simulink model "Simple_Model_Packaging_7"  (R2024a)
settings: Solver=VariableStepAuto  StartTime=0.0  StopTime=0.004  RelTol=1e-3
InitFcn:
  | Parameter_Initialize_7
undefined symbols (not defined in the file or in its folder): b, gcbh, ISDFJ_parameter, magnitude, model, n, rcfiltgaincompat, Signal_delay_length, tao, Ts
libraries: simulink x9, commdigbbndfm2 x3, commsink2 x2, commdigbbndam3 x2, commfilt2 x2, commrandsrc3 x2, commchan3 x1, commrfcorlib x1, dspsigops x1, commdigbbndcpm2 x1, commseqgen3 x1, commutil2 x1
(part 1 of 2)
settings Model: Creator=89778  LastModifiedBy=89778
settings OptimizationCC: ReuseModelBlockBuffer=off
settings RTWCC: GPUComputeCapability=3.5

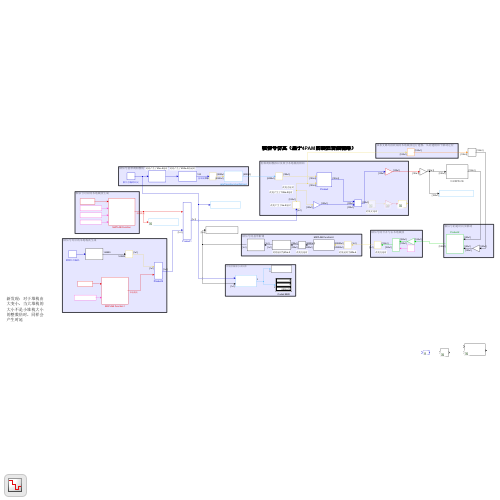
[thumbnail: Simulink's stored preview of the top-level diagram]
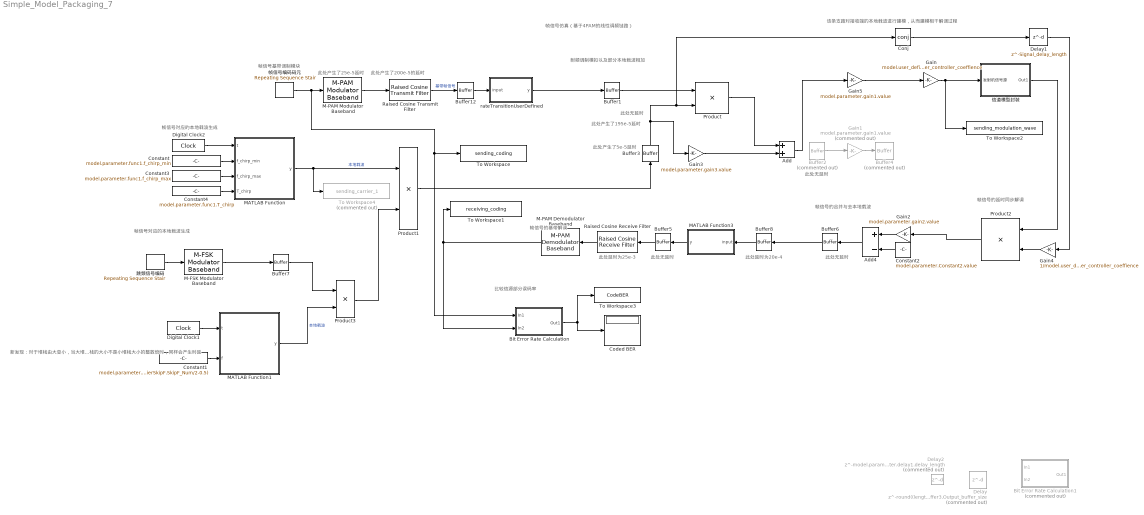
== system Simple_Model_Packaging_7 ==
  note: 帧信号的合并与去本地载波
  note: 帧信号的延时同步解调
  note: 帧信号仿真（基于4PAM的线性调频链路）
  note: 新发现：对于堆栈由大变小，当大堆栈的大小不是小堆栈大小的整数倍时，同样会产生时延
  note: 此处无延时
  note: 此处产生了25e-5延时
  note: 帧信号基带调制模块
  note: 此处产生了200e-5的延时
  note: 帧信号对应的本地载波生成
  note: 此处产生了195e-5延时
  note: 射频调制模拟以及部分本地载波相加
  note: 此处产生了5e-5延时
  note: 此处无延时
  note: 此处无延时
  note: 此处无延时
  note: 此处延时为25e-3
  note: 帧信号的基带解调
  note: 此处延时为20e-4
  note: 该条支路对接收端的本地载波进行建模，从而建模相干解调过程
  note: 比较信源部分误码率
  note: 帧信号对应的本地载波生成
  Add : Sum
  Add4 : Sum  Inputs=+-
  Bit Error Rate Calculation : Subsystem
      mask Display:
      | disp('Bit Error\nRate\nCalculation')
      | port_label('input', 1, 'Tx')
      | port_label('input', 2, 'Rx')
  Bit Error Rate Calculation1 : Subsystem  Commented=on
      mask Display:
      | disp('Bit Error\nRate\nCalculation')
      | port_label('input', 1, 'Tx')
      | port_label('input', 2, 'Rx')
  Buffer1 : Buffer  N=model.parameter.Buffer1.Output_buffer_size  OutputFrames=off
  Buffer12 : Buffer  N=model.parameter.Buffer12.Output_buffer_size  OutputFrames=off
  Buffer2 : Buffer  Commented=on  N=model.parameter.Buffer2.Output_buffer_size  OutputFrames=off
  Buffer3 : Buffer  N=model.parameter.Buffer3.Output_buffer_size  OutputFrames=off
  Buffer4 : Buffer  Commented=on  N=model.parameter.Buffer4.Output_buffer_size  OutputFrames=off
  Buffer5 : Buffer  N=model.parameter.Buffer5.Output_buffer_size  OutputFrames=off
  Buffer6 : Buffer  N=model.parameter.Buffer6.Output_buffer_size  OutputFrames=off
  Buffer7 : Buffer  N=1  OutputFrames=off
  Buffer8 : Buffer  N=model.parameter.Buffer8.Output_buffer_size  OutputFrames=off
  Coded BER : Display
  Conj : Math  Operator=conj
  Constant : Constant  Value=model.parameter.func1.f_chirp_min
  Constant1 : Constant  Value=model.parameter.CarrierSkipF.SkipF_distance*(model.parameter.CarrierSkipF.SkipF_Num/2-0.5)
  Constant2 : Constant  Value=model.parameter.Constant2.value
  Constant3 : Constant  Value=model.parameter.func1.f_chirp_max
  Constant4 : Constant  Value=model.parameter.func1.T_chirp
  Delay : Delay  Commented=on  DelayLength=round((length(model.Parameters.NoiseGen.noise_filter_b)-1)/2)-model.parameter.Buffer3.Output_buffer_size  InitialCondition=0
  Delay1 : Delay  DelayLength=Signal_delay_length  InitialCondition=0
  Delay2 : Delay  Commented=on  DelayLength=model.parameter.delay1.delay_length  InitialCondition=0  InputProcessing=Columns as channels (frame based)
  Digital Clock1 : DigitalClock  SampleTime=model.parameter.Digital_Clock2.CarrierTs
  Digital Clock2 : DigitalClock  SampleTime=model.parameter.Digital_Clock2.CarrierTs
  Gain : Gain  Gain=model.user_defined.TR.Sig_power_controller_coeffience
  Gain1 : Gain  Commented=on  Gain=model.parameter.gain1.value
  Gain2 : Gain  Gain=model.parameter.gain2.value
  Gain3 : Gain  Gain=model.parameter.gain3.value
  Gain4 : Gain  Gain=1/model.user_defined.TR.Sig_power_controller_coeffience
  Gain5 : Gain  Gain=model.parameter.gain1.value
  M-FSK Modulator Baseband : commdigbbndfm2/M-FSK Modulator Baseband  M=model.parameter.CarrierSkipF.SkipF_Num  InType=Integer  Enc=Binary  freqSep=model.parameter.CarrierSkipF.SkipF_distance  phaseType=Continuous  numSamp=ceil(model.parameter.CarrierSkipF.SkipF_time/model.parameter.Repeating_Sequence_Stair.CodeTs)*model.parameter.Raised_Cosine_Transmit_Filter.Output_samples_per_symbol  RateOptions=Enforce single-rate processing  outDataType=double
  M-PAM Demodulator Baseband : commdigbbndam3/M-PAM Demodulator Baseband  M=model.parameter.Rectangular_PAN_Demodulator_Baseband.M_Number  OutType=Integer  Dec=Gray  PowType=Min. distance between symbols  MinDist=model.parameter.Rectangular_PAM_Demodulator_Baseband.Minimum_distance  AvgPow=1  PeakPow=1  outDtype1=Inherit via internal rule  outDtype2=Inherit via internal rule  denormFactorWordLen=16  denormFactorDataTypeStr=Inherit: Same word length as input  denormFactorLastDataTypeStr=Inherit: Same word length as input  prodOutWordLen=16  prodOutRoundingMode=Floor  prodOutOverflowMode=Wrap  prodOutOvFlMode=off  prodOutOvFlModeLastStrValue=off  sumWordLen=16
  M-PAM Modulator Baseband : commdigbbndam3/M-PAM Modulator Baseband  M=model.parameter.M_PAM_Modulator_Baseband.M_ary_number  InType=Integer  Enc=Gray  PowType=Min. distance between symbols  MinDist=model.parameter.M_PAM_Modulator_Baseband.Minimum_distance  AvgPow=1  PeakPow=1  outDtype=double  outWordLen=16  outUDDataType=sfix(16)  outFracLenMode=Best precision  outFracLen=15  outDataTypeStr=double  outLastDataTypeStr=double
  MATLAB Function : MATLAB Function  InitFcn=|  TreatAsAtomicUnit=on
      | f_chirp_min=4.8e6;
      | f_chirp_max=5.2e6;
      | T_chirp=4e-4;
  MATLAB Function1 : MATLAB Function  InitFcn=|  TreatAsAtomicUnit=on
      | f_chirp_min=4.8e6;
      | f_chirp_max=5.2e6;
      | T_chirp=4e-4;
  MATLAB Function3 : MATLAB Function  TreatAsAtomicUnit=on
  Product{,1..3} (4 alike) : Product
  Raised Cosine Receive Filter : commfilt2/Raised Cosine Receive Filter  filtType=Square root  R=model.parameter.Raised_Cosine_Receive_Filter.Rolloff_factor  filtSpan=model.parameter.Raised_Cosine_Receive_Filter.Filter_span_in_symbols  N=model.parameter.Raised_Cosine_Receive_Filter.Input_samples_per_symbol  downFactor=model.parameter.Raised_Cosine_Receive_Filter.Decimation_factor  downOffset=0  filterGain=rcfiltgaincompat(gcbh)  InputProcessing=Columns as channels (frame based)  RateOptions=Enforce single-rate processing  framing=Mute  checkCoeff=off  variableName=rcRxFilt  currentFiltSpan=10  D=5  inputOffset=0  sampMode=Mute  saveAsFlag=0  rateMode=Downsampling  checkGain=Normalized  launchFVT=on  roundingMode=Floor  overflowMode=off  coeffDataTypeStr=Inherit: Same word length as input  coeffMin=[]  coeffMax=[]  coeffLastDataTypeStr=Inherit: Same word length as input  accumDataTypeStr=Inherit: Same as product output  accumLastDataTypeStr=Inherit: Same as product output  outputDataTypeStr=Inherit: Same as accumulator  outputMin=[]  outputMax=[]  outputLastDataTypeStr=Inherit: Same as accumulator
  Raised Cosine Transmit Filter : commfilt2/Raised Cosine Transmit Filter  filtType=Square root  R=model.parameter.Raised_Cosine_Transmit_Filter.Rolloff_factor  filtSpan=model.parameter.Raised_Cosine_Transmit_Filter.Filter_span_in_symbols  N=model.parameter.Raised_Cosine_Transmit_Filter.Output_samples_per_symbol  filterGain=rcfiltgaincompat(gcbh)  InputProcessing=Columns as channels (frame based)  RateOptions=Enforce single-rate processing  framing=Mute  checkCoeff=off  variableName=rcTxFilt  checkGain=Normalized  sampMode=Mute  saveAsFlag=0  currentFiltSpan=10  D=(10)/2  launchFVT=on  roundingMode=Floor  overflowMode=off  coeffDataTypeStr=Inherit: Same word length as input  coeffMin=[]  coeffMax=[]  coeffLastDataTypeStr=Inherit: Same word length as input  outputDataTypeStr=Inherit: Same as accumulator  outputMin=[]  outputMax=[]  outputLastDataTypeStr=Inherit: Same as accumulator
  To Workspace : ToWorkspace  VariableName=sending_coding  SaveFormat=Timeseries  SampleTime=-1
  To Workspace1 : ToWorkspace  VariableName=receiving_coding  SaveFormat=Timeseries  SampleTime=-1
  To Workspace2 : ToWorkspace  VariableName=sending_modulation_wave  SaveFormat=Timeseries  SampleTime=-1
  To Workspace3 : ToWorkspace  VariableName=CodeBER  SaveFormat=Timeseries  SampleTime=-1
  To Workspace4 : ToWorkspace  Commented=on  VariableName=sending_carrier_1  SaveFormat=Timeseries  SampleTime=-1
  rateTransitionUserDefined : MATLAB Function  TreatAsAtomicUnit=on
  信道模型封装 : Subsystem
  帧信号编码码元 : simulink/Sources/Repeating Sequence Stair  OutValues=model.parameter.Repeating_Sequence_Stair.output_vector  tsamp=model.parameter.Repeating_Sequence_Stair.CodeTs  OutMin=[]  OutMax=[]  OutDataTypeStr=double  OutputDataTypeScalingMode=double  OutDataType=fixdt(0,8)  ConRadixGroup=Best Precision: Vector-wise  OutScaling=2^-12
  跳频信号编码 : simulink/Sources/Repeating Sequence Stair  OutValues=model.parameter.CarrierSkipF.SkipF_vector  tsamp=model.parameter.Digital_Clock2.CarrierTs*ceil(model.parameter.CarrierSkipF.SkipF_time/model.parameter.Repeating_Sequence_Stair.CodeTs)*model.parameter.Raised_Cosine_Transmit_Filter.Output_samples_per_symbol  OutMin=[]  OutMax=[]  OutDataTypeStr=double  OutputDataTypeScalingMode=double  OutDataType=fixdt(0,8)  ConRadixGroup=Best Precision: Vector-wise  OutScaling=2^-12
  wires:
  Buffer2/1 -> Gain1/1
  Buffer12/1 -> rateTransitionUserDefined/1(input)
  rateTransitionUserDefined/1(y) -> Buffer1/1
  Raised Cosine Transmit Filter/1 -> Buffer12/1  "基带帧信号"
  M-PAM Modulator Baseband/1 -> Raised Cosine Transmit Filter/1
  Digital Clock2/1 -> MATLAB Function/1(t)
  Buffer1/1 -> Product/1
  Gain1/1 -> Buffer4/1
  Buffer5/1 -> Raised Cosine Receive Filter/1
  MATLAB Function3/1(y) -> Buffer5/1
  Buffer8/1 -> MATLAB Function3/1(input)
  Buffer6/1 -> Buffer8/1
  Raised Cosine Receive Filter/1 -> M-PAM Demodulator Baseband/1
  Constant/1 -> MATLAB Function/2(f_chirp_min)
  Constant3/1 -> MATLAB Function/3(f_chirp_max)
  Constant4/1 -> MATLAB Function/4(T_chirp)
  Gain/1 -> To Workspace2/1, 信道模型封装/1(发射机信号源)
  Gain4/1 -> Product2/2
  信道模型封装/1(Out1) -> Product2/1
  Gain3/1 -> Add/2
  Product/1 -> Add/1
  Buffer3/1 -> Gain3/1, Conj/1, Product/2
  Gain2/1 -> Add4/1
  Constant2/1 -> Add4/2
  Product2/1 -> Gain2/1
  Add4/1 -> Buffer6/1
  Add/1 -> Gain5/1
  Gain5/1 -> Gain/1
  跳频信号编码/1 -> M-FSK Modulator Baseband/1
  MATLAB Function/1(y) -> Product1/1, To Workspace4/1  "本地载波"
  Product1/1 -> Buffer3/1
  M-FSK Modulator Baseband/1 -> Buffer7/1
  Constant1/1 -> MATLAB Function1/2(f)
  Digital Clock1/1 -> MATLAB Function1/1(t)
  Buffer7/1 -> Product3/1
  MATLAB Function1/1(y) -> Product3/2  "本地载波"
  Product3/1 -> Product1/2
  M-PAM Demodulator Baseband/1 -> Bit Error Rate Calculation/2(In2), To Workspace1/1
  Bit Error Rate Calculation/1(Out1) -> Coded BER/1, To Workspace3/1
  Conj/1 -> Delay1/1
  Delay1/1 -> Gain4/1
  帧信号编码码元/1 -> Bit Error Rate Calculation/1(In1), To Workspace/1, M-PAM Modulator Baseband/1

== system Simple_Model_Packaging_7/Bit Error Rate Calculation ==
  In1 : Inport
  In2 : Inport  Port=2
  Error Rate Calculation : commsink2/Error Rate Calculation  N=920 + Signal_delay_length*4  st_delay=0  cp_mode=Entire frame  subframe=[]  PMode=Port  WsName=ErrorVec  RsMode2=off  stop=on  numErr=1e8  maxBits=1e10
  Integer to Bit Converter : simulink/Logic and Bit Operations/Integer to Bit Converter  nbits=4  signedInputValues=Unsigned  bitOrder=MSB first  outDtype=Inherit via internal rule
      settings: LibrarySourceBlock=|
      | commutil2/Integer to Bit
      | Converter
  Integer to Bit Converter1 : simulink/Logic and Bit Operations/Integer to Bit Converter  nbits=4  signedInputValues=Unsigned  bitOrder=MSB first  outDtype=Inherit via internal rule
      settings: LibrarySourceBlock=|
      | commutil2/Integer to Bit
      | Converter
  Out1 : Outport  VectorParamsAs1DForOutWhenUnconnected=off
  wires:
  Integer to Bit Converter/1 -> Error Rate Calculation/1
  Integer to Bit Converter1/1 -> Error Rate Calculation/2
  In1/1 -> Integer to Bit Converter/1
  Error Rate Calculation/1 -> Out1/1
  In2/1 -> Integer to Bit Converter1/1

== system Simple_Model_Packaging_7/Bit Error Rate Calculation1 ==
  In1 : Inport
  In2 : Inport  Port=2
  Error Rate Calculation : commsink2/Error Rate Calculation  N=920 + 4*round((length(model.Parameters.NoiseGen.noise_filter_b)-1)/2)  st_delay=0  cp_mode=Entire frame  subframe=[]  PMode=Port  WsName=ErrorVec  RsMode2=off  stop=on  numErr=1e8  maxBits=1e10
  Integer to Bit Converter : simulink/Logic and Bit Operations/Integer to Bit Converter  nbits=4  signedInputValues=Unsigned  bitOrder=MSB first  outDtype=Inherit via internal rule
      settings: LibrarySourceBlock=|
      | commutil2/Integer to Bit
      | Converter
  Integer to Bit Converter1 : simulink/Logic and Bit Operations/Integer to Bit Converter  nbits=4  signedInputValues=Unsigned  bitOrder=MSB first  outDtype=Inherit via internal rule
      settings: LibrarySourceBlock=|
      | commutil2/Integer to Bit
      | Converter
  Out1 : Outport  VectorParamsAs1DForOutWhenUnconnected=off
  wires:
  Integer to Bit Converter/1 -> Error Rate Calculation/1
  Integer to Bit Converter1/1 -> Error Rate Calculation/2
  In1/1 -> Integer to Bit Converter/1
  Error Rate Calculation/1 -> Out1/1
  In2/1 -> Integer to Bit Converter1/1

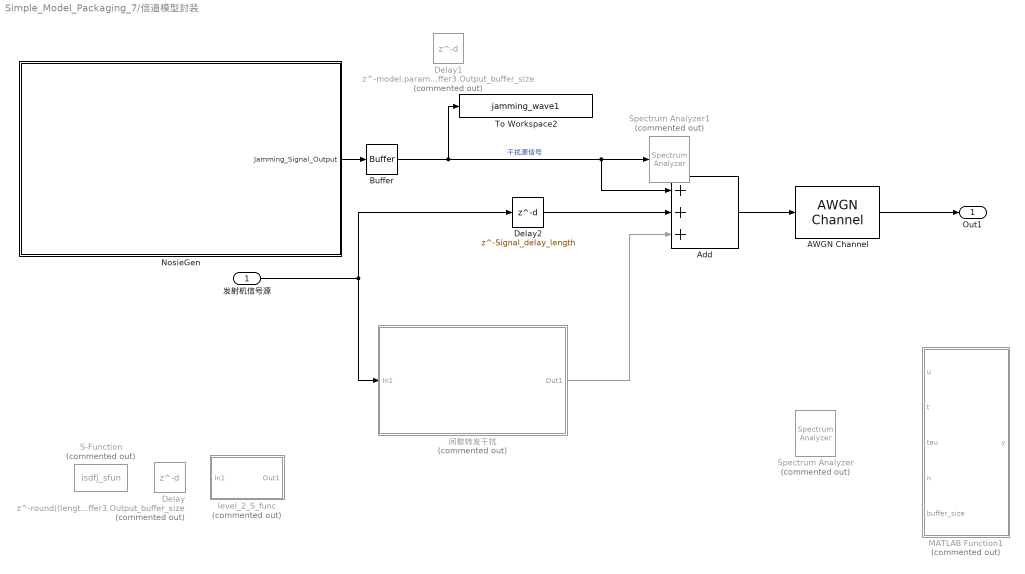
== system Simple_Model_Packaging_7/信道模型封装 ==
  发射机信号源 : Inport
  AWGN Channel : commchan3/AWGN Channel  LegacyMode=on  NoiseMethod="Signal to noise ratio  (SNR)"  noiseMode="Signal to noise ratio  (SNR)"  EbNo=10  EsNo=10  SNR=model.parameter.Awgn.SNR  BitsPerSymbol=1  SignalPower=model.parameter.Awgn.input_power  SamplesPerSymbol=1  SymbolPeriod=1  VarianceSource=Parameter  Variance=1  RandomStream=Global stream  Seed=67  SimulateUsing=Code generation
  Add : Sum  Inputs=+++
  Buffer : Buffer  N=model.parameter.Buffer1.Output_buffer_size  OutputFrames=off
  Delay : Delay  Commented=on  DelayLength=round((length(model.Parameters.NoiseGen.noise_filter_b)-1)/2)-model.parameter.Buffer3.Output_buffer_size  InitialCondition=0
  Delay1 : Delay  Commented=on  DelayLength=model.parameter.Buffer3.Output_buffer_size  InitialCondition=0
  Delay2 : Delay  DelayLength=Signal_delay_length  InitialCondition=0
  MATLAB Function1 : MATLAB Function  Commented=on  TreatAsAtomicUnit=on
  NosieGen : Subsystem
  S-Function : S-Function  Commented=on  FunctionName=isdfj_sfun  Parameters=tao,Ts,n  SFunctionDeploymentMode=off  EnableBusSupport=off
  Spectrum Analyzer : SpectrumAnalyzer  Commented=on  WindowPosition=[81 208 916 450]  SampleRate=285714285.714286  AxesScaling=Manual  Span=285714285.714286  StartFrequency=-142857142.857143  StopFrequency=142857142.857143  AveragingMethod=Exponential  YLimits=[-69.74794186129295781,48.725459434063161268]  AllowFFTLengthLessThanSamplesPerUpdate=on
  Spectrum Analyzer1 : SpectrumAnalyzer  Commented=on  WindowPosition=[746 192 916 450]  SampleRate=285714285.714286  AxesScaling=Manual  Span=285714285.714286  StartFrequency=-142857142.857143  StopFrequency=142857142.857143  AveragingMethod=Exponential  YLimits=[16.792703666476541002,24.095744456486141161]  AllowFFTLengthLessThanSamplesPerUpdate=on
  To Workspace2 : ToWorkspace  VariableName=jamming_wave1  SaveFormat=Timeseries  SampleTime=-1
  level_2_S_func : Subsystem  Commented=on
  间歇转发干扰 : Subsystem  Commented=on
  Out1 : Outport
  wires:
  AWGN Channel/1 -> Out1/1
  Add/1 -> AWGN Channel/1
  发射机信号源/1 -> Delay2/1, 间歇转发干扰/1(In1)
  Buffer/1 -> To Workspace2/1, Spectrum Analyzer1/1, Add/1  "干扰源信号"
  NosieGen/1(Jamming_Signal_Output) -> Buffer/1
  Delay2/1 -> Add/2
  间歇转发干扰/1(Out1) -> Add/3

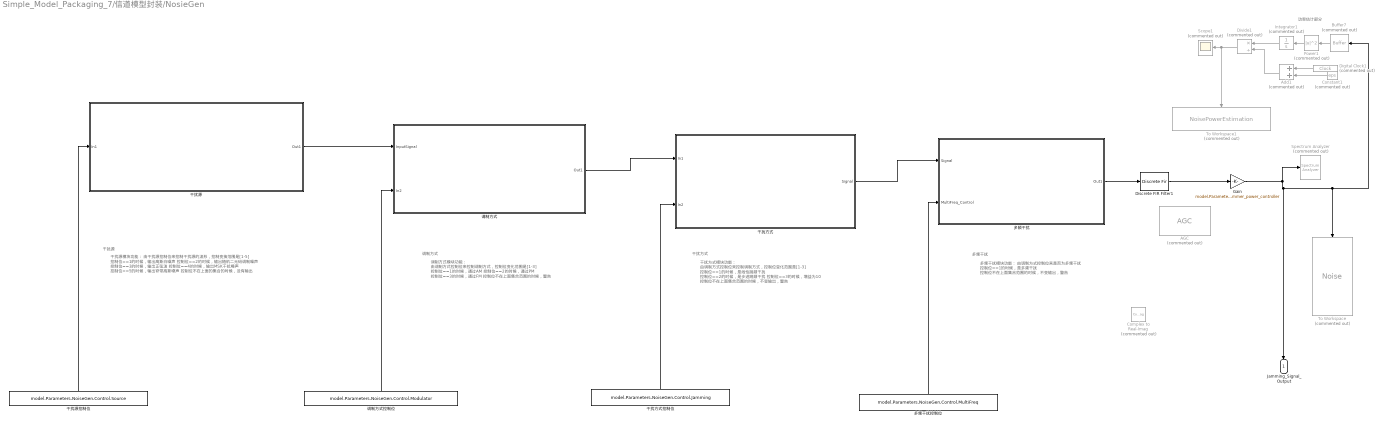
== system Simple_Model_Packaging_7/信道模型封装/NosieGen ==
  note: 调制方式
  note: 调制方式模块功能：
      | 由调制方式控制位来控制调制方式，控制位变化范围是[1-3]
      | 控制位==1的时候，通过AM
      | 控制位==2的时候，通过PM
      | 控制位==3的时候，通过FM
      |
      | 控制位不在上面集合范围的时候，警告
  note: 干扰方式模块功能：
      | 由调制方式控制位来控制调制方式，控制位变化范围是[1-3]
      | 控制位==1的时候，是线性跳频干扰
      | 控制位==2的时候，是步进跳频干扰
      | 控制位==3的时候，增益为10
      |
      | 控制位不在上面集合范围的时候，不变输出，警告
  note: 干扰源
  note: 功率估计部分
  note: 干扰方式
  note: 干扰源模块功能：
      | 由干扰源控制位来控制干扰源的波形，控制变换范围是[1-5]
      | 控制位==1的时候，输出高斯白噪声
      | 控制位==2的时候，输出随机二元码调制噪声
      | 控制位==3的时候，输出正弦波
      | 控制位==4的时候，输出MSK干扰噪声
      | 控制位==5的时候，输出窄带高斯噪声
      | 控制位不在上面的集合的时候，没有输出
  note: 多频干扰模块功能：
      | 由调制方式控制位来是否为多频干扰
      | 控制位==1的时候，是多频干扰
      |
      | 控制位不在上面集合范围的时候，不变输出，警告
  note: 多频干扰
  AGC : commrfcorlib/AGC  Commented=on  LegacyMode=off  DetectorMethod=Rectifier  LoopMethod=Linear  UpdatePeriod=100  StepSize=0.1  AdaptationStepSize=0.01  DesiredOutputPower=1  AveragingLength=100  MaximumGain=30  MaxPowerGain=60  GainOutputPort=off  InputPowerOutputPort=off  SimulateUsing=Interpreted execution
  Add1 : Sum  Commented=on
  Buffer7 : Buffer  Commented=on  N=1  OutputFrames=off
  Complex to Real-Imag : ComplexToRealImag  Commented=on
  Constant1 : Constant  Commented=on  Value=eps  SampleTime=model.Parameters.NoiseGen.NoiseTs
  Digital Clock1 : DigitalClock  Commented=on  SampleTime=model.Parameters.NoiseGen.NoiseTs
  Discrete FIR Filter1 : DiscreteFir  Coefficients=model.Parameters.NoiseGen.noise_filter_b
  Divide1 : Product  Commented=on  Inputs=*/
  Gain : Gain  Gain=model.Parameters.jammer_power_controller
  Integrator1 : Integrator  Commented=on
  Power1 : Math  Commented=on  Operator=magnitude^2
  Scope1 : Scope  Commented=on
  Spectrum Analyzer : SpectrumAnalyzer  Commented=on  WindowPosition=[162 288 916 450]  SampleRate=340000000  AxesScaling=Manual  Span=340000000  StartFrequency=-170000000  StopFrequency=170000000  AveragingMethod=Exponential  YLimits=[16.792703666476541002,24.095744456486141161]  AllowFFTLengthLessThanSamplesPerUpdate=on
  To Workspace : ToWorkspace  Commented=on  VariableName=Noise  SaveFormat=Timeseries  SampleTime=-1
  To Workspace1 : ToWorkspace  Commented=on  VariableName=NoisePowerEstimation  SaveFormat=Timeseries  SampleTime=-1
  多频干扰 : Subsystem
  多频干扰控制位 : Constant  Value=model.Parameters.NoiseGen.Control.MultiFreq  SampleTime=Inf
  干扰方式 : Subsystem
  干扰方式控制位 : Constant  Value=model.Parameters.NoiseGen.Control.Jamming  SampleTime=Inf
  干扰源 : Subsystem
  干扰源控制位 : Constant  Value=model.Parameters.NoiseGen.Control.Source  SampleTime=Inf
  调制方式 : Subsystem
  调制方式控制位 : Constant  Value=model.Parameters.NoiseGen.Control.Modulator  SampleTime=Inf
  Jamming_Signal_Output : Outport
  wires:
  Integrator1/1 -> Divide1/1
  Power1/1 -> Integrator1/1
  干扰方式控制位/1 -> 干扰方式/2(In2)
  调制方式控制位/1 -> 调制方式/2(In2)
  Digital Clock1/1 -> Add1/1
  Divide1/1 -> Scope1/1, To Workspace1/1
  干扰源控制位/1 -> 干扰源/1(In1)
  Constant1/1 -> Add1/2
  Add1/1 -> Divide1/2
  Buffer7/1 -> Power1/1
  Gain/1 -> Jamming_Signal_Output/1, Buffer7/1, To Workspace/1, Spectrum Analyzer/1
  调制方式/1(Out1) -> 干扰方式/1(In1)
  干扰源/1(Out1) -> 调制方式/1(InputSignal)
  多频干扰控制位/1 -> 多频干扰/2(MultiFreq_Control)
  干扰方式/1(Signal) -> 多频干扰/1(Signal)
  多频干扰/1(Out1) -> Discrete FIR Filter1/1
  Discrete FIR Filter1/1 -> Gain/1

== system Simple_Model_Packaging_7/信道模型封装/level_2_S_func ==
  In1 : Inport
  Buffer1 : Buffer  N=1  OutputFrames=off
  Buffer2 : Buffer  N=100  OutputFrames=off
  Level-2 MATLAB S-Function : M-S-Function  FunctionName=isdfj_sfun  Parameters=2e-6, 10e-6, 1
  Out1 : Outport
  wires:
  Level-2 MATLAB S-Function/1 -> Buffer2/1
  Buffer2/1 -> Out1/1
  Buffer1/1 -> Level-2 MATLAB S-Function/1
  In1/1 -> Buffer1/1

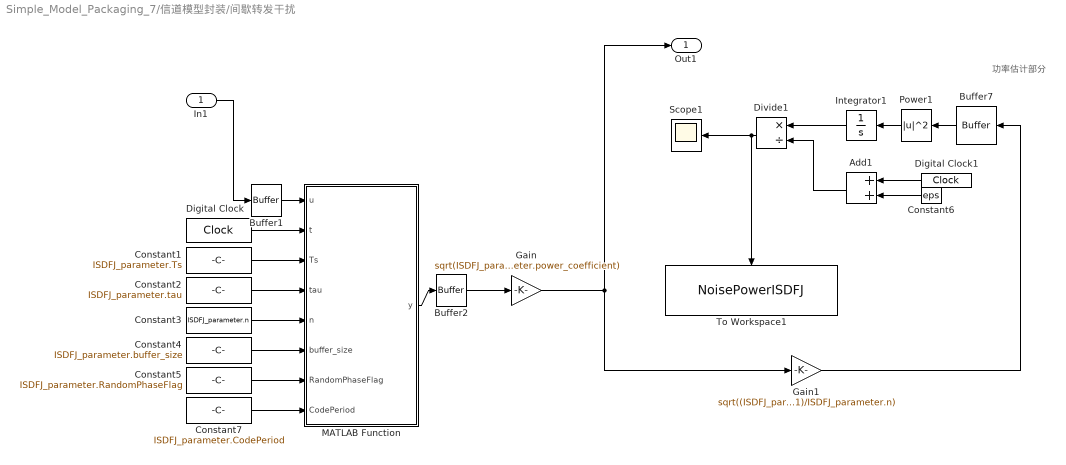
== system Simple_Model_Packaging_7/信道模型封装/间歇转发干扰 ==
  note: 功率估计部分
  In1 : Inport
  Add1 : Sum
  Buffer1 : Buffer  N=1  OutputFrames=off
  Buffer2 : Buffer  N=100  OutputFrames=off
  Buffer7 : Buffer  N=1  OutputFrames=off
  Constant1 : Constant  Value=ISDFJ_parameter.Ts
  Constant2 : Constant  Value=ISDFJ_parameter.tau
  Constant3 : Constant  Value=ISDFJ_parameter.n
  Constant4 : Constant  Value=ISDFJ_parameter.buffer_size
  Constant5 : Constant  Value=ISDFJ_parameter.RandomPhaseFlag
  Constant6 : Constant  Value=eps  SampleTime=model.Parameters.NoiseGen.NoiseTs
  Constant7 : Constant  Value=ISDFJ_parameter.CodePeriod
  Digital Clock : DigitalClock  SampleTime=model.Parameters.NoiseGen.NoiseTs
  Digital Clock1 : DigitalClock  SampleTime=model.Parameters.NoiseGen.NoiseTs
  Divide1 : Product  Inputs=*/
  Gain : Gain  Gain=sqrt(ISDFJ_parameter.power_coefficient)
  Gain1 : Gain  Gain=sqrt((ISDFJ_parameter.n+1)/ISDFJ_parameter.n)
  Integrator1 : Integrator
  MATLAB Function : MATLAB Function  TreatAsAtomicUnit=on
  Power1 : Math  Operator=magnitude^2
  Scope1 : Scope
  To Workspace1 : ToWorkspace  VariableName=NoisePowerISDFJ  SaveFormat=Timeseries  SampleTime=-1
  Out1 : Outport
  wires:
  Constant2/1 -> MATLAB Function/4(tau)
  In1/1 -> Buffer1/1
  Constant1/1 -> MATLAB Function/3(Ts)
  Constant3/1 -> MATLAB Function/5(n)
  Digital Clock/1 -> MATLAB Function/2(t)
  MATLAB Function/1(y) -> Buffer2/1
  Constant4/1 -> MATLAB Function/6(buffer_size)
  Buffer1/1 -> MATLAB Function/1(u)
  Constant5/1 -> MATLAB Function/7(RandomPhaseFlag)
  Power1/1 -> Integrator1/1
  Add1/1 -> Divide1/2
  Buffer7/1 -> Power1/1
  Constant6/1 -> Add1/2
  Integrator1/1 -> Divide1/1
  Digital Clock1/1 -> Add1/1
  Divide1/1 -> Scope1/1, To Workspace1/1
  Constant7/1 -> MATLAB Function/8(CodePeriod)
  Gain/1 -> Out1/1, Gain1/1
  Gain1/1 -> Buffer7/1
  Buffer2/1 -> Gain/1

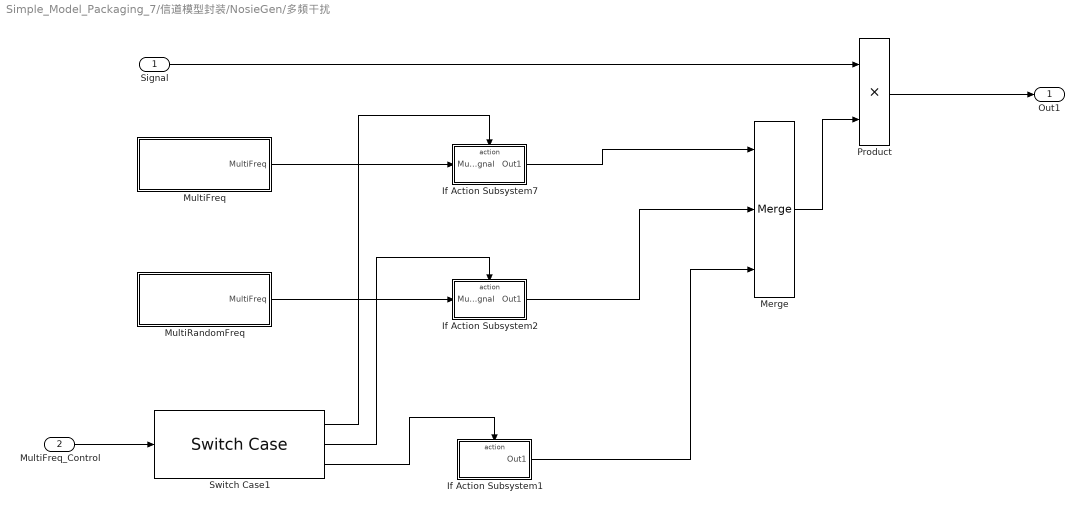
== system Simple_Model_Packaging_7/信道模型封装/NosieGen/多频干扰 ==
  Signal : Inport
  MultiFreq_Control : Inport  Port=2
  If Action Subsystem1 : Subsystem  TreatAsAtomicUnit=on
  If Action Subsystem2 : Subsystem  TreatAsAtomicUnit=on
  If Action Subsystem7 : Subsystem  TreatAsAtomicUnit=on
  Merge : Merge  Inputs=3
  MultiFreq : Subsystem
  MultiRandomFreq : Subsystem
  Product : Product
  Switch Case1 : SwitchCase  CaseConditions={1,2}
  Out1 : Outport
  wires:
  Switch Case1/3 -> If Action Subsystem1/Action
  Signal/1 -> Product/1
  MultiFreq_Control/1 -> Switch Case1/1
  Merge/1 -> Product/2
  Product/1 -> Out1/1
  Switch Case1/1 -> If Action Subsystem7/Action
  MultiFreq/1(MultiFreq) -> If Action Subsystem7/1(MultiFreqSignal)
  If Action Subsystem7/1(Out1) -> Merge/1
  If Action Subsystem1/1(Out1) -> Merge/3
  MultiRandomFreq/1(MultiFreq) -> If Action Subsystem2/1(MultiRandomFreqSignal)
  Switch Case1/2 -> If Action Subsystem2/Action
  If Action Subsystem2/1(Out1) -> Merge/2

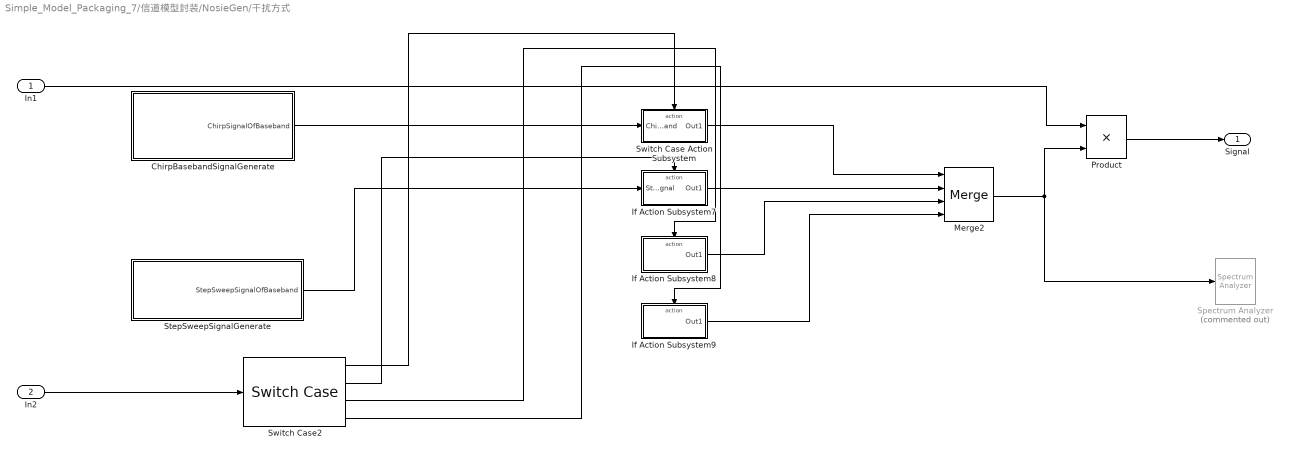
== system Simple_Model_Packaging_7/信道模型封装/NosieGen/干扰方式 ==
  In1 : Inport
  In2 : Inport  Port=2
  ChirpBasebandSignalGenerate : Subsystem
      settings: AttributesFormatString=|
      | 线性调频模块：线性调频公式(y=exp(2*pi*(f_min*t+0.5*k_chirp*t^2)))
      | 输入参数：
      | 1. f_min,为线性调频信号的起始频率
      | 2.f_max为线性调频信号的终止频率
      | 3.T_chirp为线性调频信号的调频时间
      | 斜率k_sweep = (f_min-f_max)/T_chirp
  If Action Subsystem7 : Subsystem  TreatAsAtomicUnit=on
  If Action Subsystem8 : Subsystem  TreatAsAtomicUnit=on
  If Action Subsystem9 : Subsystem  TreatAsAtomicUnit=on
  Merge2 : Merge  Inputs=4
  Product : Product
  Spectrum Analyzer : SpectrumAnalyzer  Commented=on  WindowPosition=[-1041 199 916 450]  SampleRate=340000000  AxesScaling=Manual  Span=340000000  StartFrequency=-170000000  StopFrequency=170000000  AveragingMethod=Exponential  YLimits=[-55.253534235882824532,34.529267970454846193]  AllowFFTLengthLessThanSamplesPerUpdate=on
  StepSweepSignalGenerate : Subsystem
  Switch Case Action Subsystem : Subsystem  TreatAsAtomicUnit=on
  Switch Case2 : SwitchCase  CaseConditions={1,2,3}
  Signal : Outport
  wires:
  If Action Subsystem9/1(Out1) -> Merge2/4
  Switch Case Action Subsystem/1(Out1) -> Merge2/1
  If Action Subsystem8/1(Out1) -> Merge2/3
  Switch Case2/3 -> If Action Subsystem8/Action
  Switch Case2/1 -> Switch Case Action Subsystem/Action
  Switch Case2/2 -> If Action Subsystem7/Action
  Switch Case2/4 -> If Action Subsystem9/Action
  ChirpBasebandSignalGenerate/1(ChirpSignalOfBaseband) -> Switch Case Action Subsystem/1(ChirpSignalOfBaseband)
  If Action Subsystem7/1(Out1) -> Merge2/2
  Merge2/1 -> Spectrum Analyzer/1, Product/2
  Product/1 -> Signal/1
  In1/1 -> Product/1
  In2/1 -> Switch Case2/1
  StepSweepSignalGenerate/1(StepSweepSignalOfBaseband) -> If Action Subsystem7/1(StepSweepSignal)

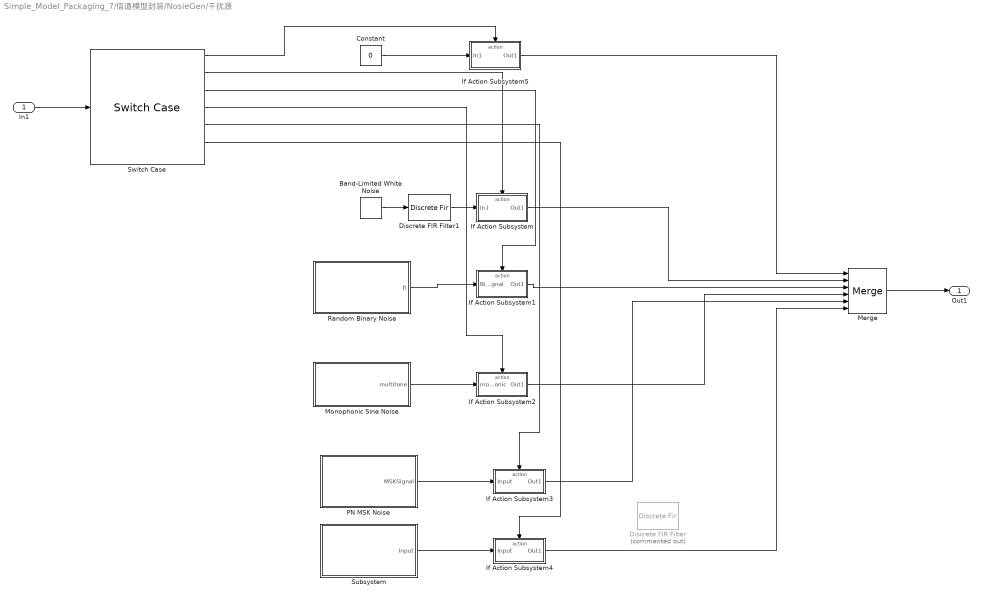
== system Simple_Model_Packaging_7/信道模型封装/NosieGen/干扰源 ==
  In1 : Inport
  Band-Limited White Noise : simulink/Sources/Band-Limited White Noise  Cov=model.Parameters.NoiseGen.GaussPower  Ts=model.Parameters.NoiseGen.NoiseTs  seed=model.Parameters.NoiseGen.GaussSeed
  Constant : Constant  Value=0  SampleTime=model.Parameters.NoiseGen.NoiseTs
  Discrete FIR Filter : DiscreteFir  Commented=on  Coefficients=b
  Discrete FIR Filter1 : DiscreteFir  Coefficients=model.Parameters.NoiseGen.pulse_noise_filter_b
  If Action Subsystem : Subsystem  TreatAsAtomicUnit=on
  If Action Subsystem1 : Subsystem  TreatAsAtomicUnit=on
  If Action Subsystem2 : Subsystem  TreatAsAtomicUnit=on
  If Action Subsystem3 : Subsystem  TreatAsAtomicUnit=on
  If Action Subsystem4 : Subsystem  TreatAsAtomicUnit=on
  If Action Subsystem5 : Subsystem  TreatAsAtomicUnit=on
  Merge : Merge  Inputs=6
  Monophonic Sine Noise : Subsystem
  PN MSK Noise : Subsystem
  Random Binary Noise : Subsystem
  Subsystem : Subsystem
  Switch Case : SwitchCase  CaseConditions={0,1,2,3,4,5}
  Out1 : Outport
  wires:
  Switch Case/3 -> If Action Subsystem1/Action
  If Action Subsystem2/1(Out1) -> Merge/4
  Band-Limited White Noise/1 -> Discrete FIR Filter1/1
  If Action Subsystem1/1(Out1) -> Merge/3
  Random Binary Noise/1(Jt) -> If Action Subsystem1/1(Binary_Random_Signal)
  Switch Case/4 -> If Action Subsystem2/Action
  Switch Case/2 -> If Action Subsystem/Action
  Merge/1 -> Out1/1
  In1/1 -> Switch Case/1
  Monophonic Sine Noise/1(multitone) -> If Action Subsystem2/1(monophonic)
  Switch Case/5 -> If Action Subsystem3/Action
  If Action Subsystem3/1(Out1) -> Merge/5
  If Action Subsystem/1(Out1) -> Merge/2
  PN MSK Noise/1(MSKSignal) -> If Action Subsystem3/1(Input)
  Switch Case/6 -> If Action Subsystem4/Action
  Subsystem/1(Input) -> If Action Subsystem4/1(Input)
  If Action Subsystem4/1(Out1) -> Merge/6
  Switch Case/1 -> If Action Subsystem5/Action
  Constant/1 -> If Action Subsystem5/1(In1)
  If Action Subsystem5/1(Out1) -> Merge/1
  Discrete FIR Filter1/1 -> If Action Subsystem/1(In1)

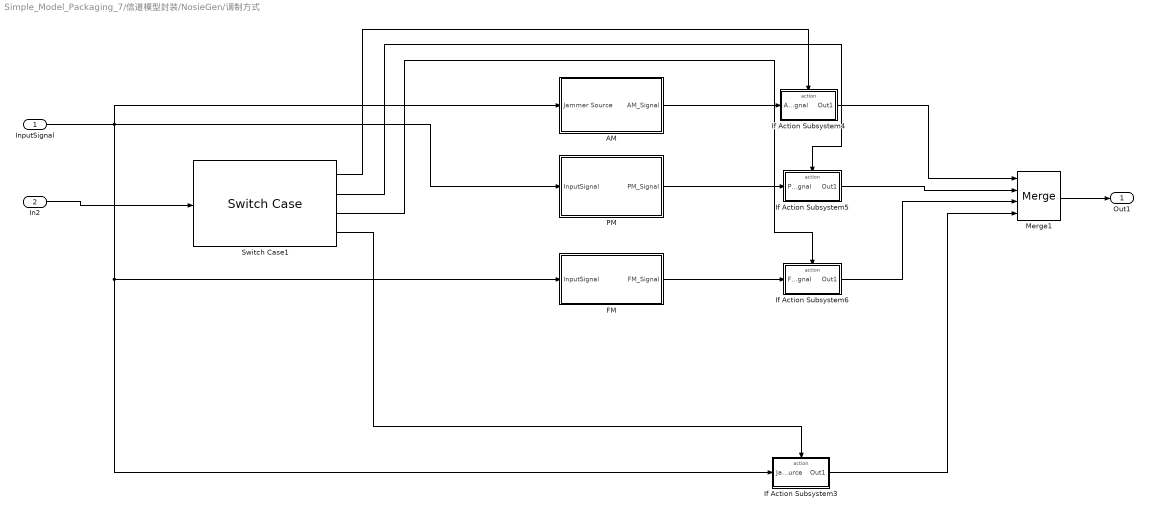
== system Simple_Model_Packaging_7/信道模型封装/NosieGen/调制方式 ==
  InputSignal : Inport
  In2 : Inport  Port=2
  AM : Subsystem
  FM : Subsystem
  If Action Subsystem3 : Subsystem  TreatAsAtomicUnit=on
  If Action Subsystem4 : Subsystem  TreatAsAtomicUnit=on
  If Action Subsystem5 : Subsystem  TreatAsAtomicUnit=on
  If Action Subsystem6 : Subsystem  TreatAsAtomicUnit=on
  Merge1 : Merge  Inputs=4
  PM : Subsystem
  Switch Case1 : SwitchCase  CaseConditions={1,2,3}
  Out1 : Outport
  wires:
  In2/1 -> Switch Case1/1
  PM/1(PM_Signal) -> If Action Subsystem5/1(PM_Signal)
  Merge1/1 -> Out1/1
  If Action Subsystem3/1(Out1) -> Merge1/4
  If Action Subsystem6/1(Out1) -> Merge1/3
  If Action Subsystem5/1(Out1) -> Merge1/2
  InputSignal/1 -> FM/1(InputSignal), If Action Subsystem3/1(Jammer Source), PM/1(InputSignal), AM/1(Jammer Source)
  AM/1(AM_Signal) -> If Action Subsystem4/1(AM_Signal)
  Switch Case1/2 -> If Action Subsystem5/Action
  Switch Case1/3 -> If Action Subsystem6/Action
  Switch Case1/1 -> If Action Subsystem4/Action
  If Action Subsystem4/1(Out1) -> Merge1/1
  FM/1(FM_Signal) -> If Action Subsystem6/1(FM_Signal)
  Switch Case1/4 -> If Action Subsystem3/Action

== system Simple_Model_Packaging_7/信道模型封装/NosieGen/多频干扰/If Action Subsystem1 ==
  Action Port : ActionPort  ActionPortLabel=default:
  Constant : Constant
  Constant1 : Constant  Value=0
  Real-Imag to Complex : RealImagToComplex
  Out1 : Outport
  wires:
  Constant/1 -> Real-Imag to Complex/1
  Real-Imag to Complex/1 -> Out1/1
  Constant1/1 -> Real-Imag to Complex/2

== system Simple_Model_Packaging_7/信道模型封装/NosieGen/多频干扰/If Action Subsystem2 ==
  MultiRandomFreqSignal : Inport
  Action Port : ActionPort  ActionPortLabel=case [ 2 ]:
  Out1 : Outport
  wires:
  MultiRandomFreqSignal/1 -> Out1/1

== system Simple_Model_Packaging_7/信道模型封装/NosieGen/多频干扰/If Action Subsystem7 ==
  MultiFreqSignal : Inport
  Action Port : ActionPort  ActionPortLabel=case [ 1 ]:
  Out1 : Outport
  wires:
  MultiFreqSignal/1 -> Out1/1

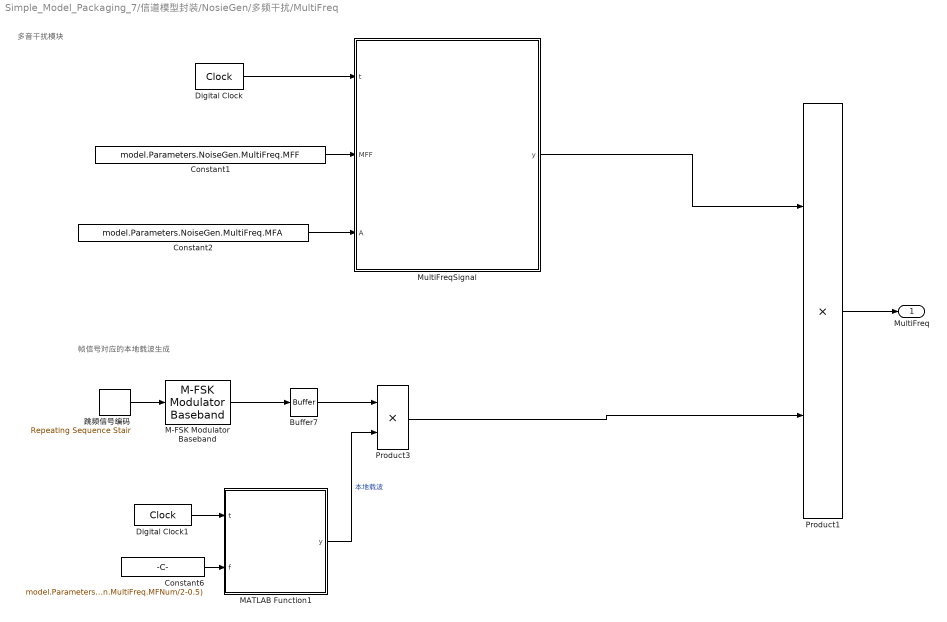
== system Simple_Model_Packaging_7/信道模型封装/NosieGen/多频干扰/MultiFreq ==
  note: 多音干扰模块
  note: 帧信号对应的本地载波生成
  Buffer7 : Buffer  N=1  OutputFrames=off
  Constant1 : Constant  Value=model.Parameters.NoiseGen.MultiFreq.MFF
  Constant2 : Constant  Value=model.Parameters.NoiseGen.MultiFreq.MFA
  Constant6 : Constant  Value=model.Parameters.NoiseGen.MultiFreq.MFDistance*(model.Parameters.NoiseGen.MultiFreq.MFNum/2-0.5)
  Digital Clock : DigitalClock  SampleTime=model.Parameters.NoiseGen.NoiseTs
  Digital Clock1 : DigitalClock  SampleTime=model.Parameters.NoiseGen.NoiseTs
  M-FSK Modulator Baseband : commdigbbndfm2/M-FSK Modulator Baseband  M=model.Parameters.NoiseGen.MultiFreq.MFNum  InType=Integer  Enc=Binary  freqSep=model.Parameters.NoiseGen.MultiFreq.MFDistance  phaseType=Continuous  numSamp=ceil(model.Parameters.NoiseGen.MultiFreq.MFTime/model.Parameters.NoiseGen.NoiseTs)  RateOptions=Enforce single-rate processing  outDataType=double
  MATLAB Function1 : MATLAB Function  InitFcn=|  TreatAsAtomicUnit=on
      | f_chirp_min=4.8e6;
      | f_chirp_max=5.2e6;
      | T_chirp=4e-4;
  MultiFreqSignal : MATLAB Function  TreatAsAtomicUnit=on
  Product1 : Product
  Product3 : Product
  跳频信号编码 : simulink/Sources/Repeating Sequence Stair  OutValues=model.Parameters.NoiseGen.MultiFreq.MFSequence  tsamp=model.Parameters.NoiseGen.NoiseTs*ceil(model.Parameters.NoiseGen.MultiFreq.MFTime/model.Parameters.NoiseGen.NoiseTs)  OutMin=[]  OutMax=[]  OutDataTypeStr=double  OutputDataTypeScalingMode=double  OutDataType=fixdt(0,8)  ConRadixGroup=Best Precision: Vector-wise  OutScaling=2^-12
  MultiFreq : Outport
  wires:
  Constant1/1 -> MultiFreqSignal/2(MFF)
  MultiFreqSignal/1(y) -> Product1/1
  Product1/1 -> MultiFreq/1
  Digital Clock/1 -> MultiFreqSignal/1(t)
  Constant2/1 -> MultiFreqSignal/3(A)
  Digital Clock1/1 -> MATLAB Function1/1(t)
  Buffer7/1 -> Product3/1
  跳频信号编码/1 -> M-FSK Modulator Baseband/1
  M-FSK Modulator Baseband/1 -> Buffer7/1
  MATLAB Function1/1(y) -> Product3/2  "本地载波"
  Constant6/1 -> MATLAB Function1/2(f)
  Product3/1 -> Product1/2

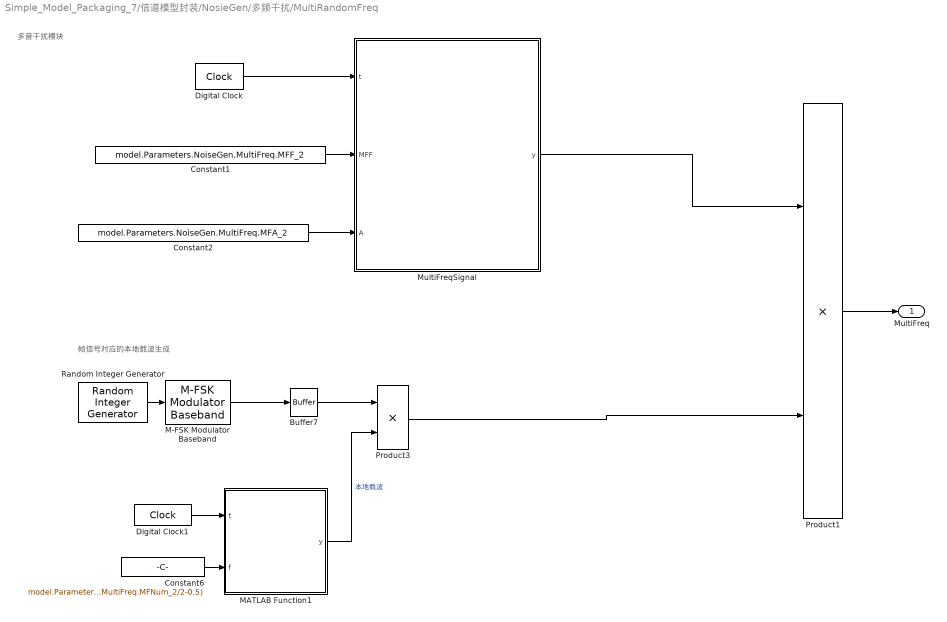
== system Simple_Model_Packaging_7/信道模型封装/NosieGen/多频干扰/MultiRandomFreq ==
  note: 帧信号对应的本地载波生成
  note: 多音干扰模块
  Buffer7 : Buffer  N=1  OutputFrames=off
  Constant1 : Constant  Value=model.Parameters.NoiseGen.MultiFreq.MFF_2
  Constant2 : Constant  Value=model.Parameters.NoiseGen.MultiFreq.MFA_2
  Constant6 : Constant  Value=model.Parameters.NoiseGen.MultiFreq.MFDistance_2*(model.Parameters.NoiseGen.MultiFreq.MFNum_2/2-0.5)
  Digital Clock : DigitalClock  SampleTime=model.Parameters.NoiseGen.NoiseTs
  Digital Clock1 : DigitalClock  SampleTime=model.Parameters.NoiseGen.NoiseTs
  M-FSK Modulator Baseband : commdigbbndfm2/M-FSK Modulator Baseband  M=model.Parameters.NoiseGen.MultiFreq.MFNum_2  InType=Integer  Enc=Binary  freqSep=model.Parameters.NoiseGen.MultiFreq.MFDistance_2  phaseType=Continuous  numSamp=ceil(model.Parameters.NoiseGen.MultiFreq.MFTime_2/model.Parameters.NoiseGen.NoiseTs)  RateOptions=Enforce single-rate processing  outDataType=double
  MATLAB Function1 : MATLAB Function  InitFcn=|  TreatAsAtomicUnit=on
      | f_chirp_min=4.8e6;
      | f_chirp_max=5.2e6;
      | T_chirp=4e-4;
  MultiFreqSignal : MATLAB Function  TreatAsAtomicUnit=on
  Product1 : Product
  Product3 : Product
  Random Integer Generator : commrandsrc3/Random Integer Generator  SetSize=model.Parameters.NoiseGen.MultiFreq.MF_2  SeedSource=Auto  Seed=0  SampleTime=model.Parameters.NoiseGen.NoiseTs*ceil(model.Parameters.NoiseGen.MultiFreq.MFTime_2/model.Parameters.NoiseGen.NoiseTs)  SamplesPerFrame=1  OutputDataType=double  SimulateUsing=Interpreted execution
  MultiFreq : Outport
  wires:
  Product3/1 -> Product1/2
  Constant6/1 -> MATLAB Function1/2(f)
  MATLAB Function1/1(y) -> Product3/2  "本地载波"
  M-FSK Modulator Baseband/1 -> Buffer7/1
  Buffer7/1 -> Product3/1
  Digital Clock1/1 -> MATLAB Function1/1(t)
  Constant2/1 -> MultiFreqSignal/3(A)
  Digital Clock/1 -> MultiFreqSignal/1(t)
  Product1/1 -> MultiFreq/1
  MultiFreqSignal/1(y) -> Product1/1
  Constant1/1 -> MultiFreqSignal/2(MFF)
  Random Integer Generator/1 -> M-FSK Modulator Baseband/1

== system Simple_Model_Packaging_7/信道模型封装/NosieGen/干扰方式/ChirpBasebandSignalGenerate ==
  note: 线性调频模块：线性调频公式(y=exp(2*pi*(fmin*t+0.5*k_chirp*t^2)))
      | 输入参数：
      | 1.fmin,为线性调频信号的起始频率
      | 2.fmax为线性调频信号的终止频率
      | 3.T_chirp为线性调频信号的调频时间
      | 斜率k_sweep = (f_min-f_max)/T_chirp
  note: 线性调频模块
  Chirp_Signal_Generation : MATLAB Function  TreatAsAtomicUnit=on
  Constant : Constant  Value=model.Parameters.NoiseGen.Jamming.LinearSweepFmin
  Constant1 : Constant  Value=model.Parameters.NoiseGen.Jamming.LinearSweepT
  Constant2 : Constant  Value=model.Parameters.NoiseGen.Jamming.LinearSweepK
  Digital Clock : DigitalClock  SampleTime=model.Parameters.NoiseGen.NoiseTs
  Frequency_Check : Subsystem  Commented=on
  ChirpSignalOfBaseband : Outport
  wires:
  Digital Clock/1 -> Chirp_Signal_Generation/1(t)
  Chirp_Signal_Generation/1(y) -> ChirpSignalOfBaseband/1  "ChirpSignal"
  Frequency_Check/1(FrequencyConversionLine) -> ?
  Constant/1 -> Chirp_Signal_Generation/2(f_chirp_min)
  Constant2/1 -> Chirp_Signal_Generation/4(k_chirp)
  Constant1/1 -> Chirp_Signal_Generation/3(T_chirp)

== system Simple_Model_Packaging_7/信道模型封装/NosieGen/干扰方式/If Action Subsystem7 ==
  StepSweepSignal : Inport
  Action Port : ActionPort  ActionPortLabel=case [ 2 ]:
  Out1 : Outport
  wires:
  StepSweepSignal/1 -> Out1/1

== system Simple_Model_Packaging_7/信道模型封装/NosieGen/干扰方式/If Action Subsystem8 ==
  Action Port : ActionPort  ActionPortLabel=case [ 3 ]:
  Constant : Constant  Value=10
  Constant1 : Constant  Value=0
  Real-Imag to Complex : RealImagToComplex
  Out1 : Outport
  wires:
  Constant/1 -> Real-Imag to Complex/1
  Real-Imag to Complex/1 -> Out1/1
  Constant1/1 -> Real-Imag to Complex/2

== system Simple_Model_Packaging_7/信道模型封装/NosieGen/干扰方式/If Action Subsystem9 ==
  Action Port : ActionPort  ActionPortLabel=default:
  Constant : Constant
  Constant1 : Constant  Value=0
  Real-Imag to Complex : RealImagToComplex
  Out1 : Outport
  wires:
  Constant/1 -> Real-Imag to Complex/1
  Real-Imag to Complex/1 -> Out1/1
  Constant1/1 -> Real-Imag to Complex/2

== system Simple_Model_Packaging_7/信道模型封装/NosieGen/干扰方式/StepSweepSignalGenerate ==
  note: 步进调频模块
  note: 新发现：对于堆栈由大变小，当大堆栈的大小不是小堆栈大小的整数倍时，同样会产生时延
  Constant : Constant  Value=model.Parameters.NoiseGen.NoiseTs
  Constant1 : Constant  Value=model.Parameters.NoiseGen.Jamming.StepSweepFmin
  Constant2 : Constant  Value=model.Parameters.NoiseGen.Jamming.StepSweepT
  Constant3 : Constant  Value=model.Parameters.NoiseGen.Jamming.StepSweepDeltaFstep
  Constant4 : Constant  Value=model.Parameters.NoiseGen.Jamming.StepSweepTDwell
  Constant5 : Constant  Value=model.Parameters.NoiseGen.Jamming.StepSweepN
  Digital Clock : DigitalClock  SampleTime=model.Parameters.NoiseGen.NoiseTs
  StepSweep_Signal : MATLAB Function  TreatAsAtomicUnit=on
  StepSweepSignalOfBaseband : Outport
  wires:
  Digital Clock/1 -> StepSweep_Signal/1(t)
  Constant/1 -> StepSweep_Signal/6(Ts)
  Constant1/1 -> StepSweep_Signal/2(f_stepSweep_min)
  Constant2/1 -> StepSweep_Signal/3(T_stepSweep)
  Constant3/1 -> StepSweep_Signal/4(delta_f_stepSweep)
  Constant4/1 -> StepSweep_Signal/5(T_stepSweep_dwell)
  Constant5/1 -> StepSweep_Signal/7(N_stepSweep)
  StepSweep_Signal/1(y) -> StepSweepSignalOfBaseband/1  "StepSweepSignal"

== system Simple_Model_Packaging_7/信道模型封装/NosieGen/干扰方式/Switch Case Action Subsystem ==
  ChirpSignalOfBaseband : Inport
  Action Port : ActionPort  ActionPortLabel=case [ 1 ]:
  Out1 : Outport
  wires:
  ChirpSignalOfBaseband/1 -> Out1/1

== system Simple_Model_Packaging_7/信道模型封装/NosieGen/干扰源/If Action Subsystem ==
  In1 : Inport
  Action Port : ActionPort  ActionPortLabel=case [ 1 ]:
  Out1 : Outport
  wires:
  In1/1 -> Out1/1

== system Simple_Model_Packaging_7/信道模型封装/NosieGen/干扰源/If Action Subsystem1 ==
  Binary_Random_Signal : Inport
  Action Port : ActionPort  ActionPortLabel=case [ 2 ]:
  Out1 : Outport
  wires:
  Binary_Random_Signal/1 -> Out1/1

== system Simple_Model_Packaging_7/信道模型封装/NosieGen/干扰源/If Action Subsystem2 ==
  monophonic : Inport
  Action Port : ActionPort  ActionPortLabel=case [ 3 ]:
  Out1 : Outport
  wires:
  monophonic/1 -> Out1/1

== system Simple_Model_Packaging_7/信道模型封装/NosieGen/干扰源/If Action Subsystem3 ==
  Input : Inport
  Action Port : ActionPort  ActionPortLabel=case [ 4 ]:
  Out1 : Outport
  wires:
  Input/1 -> Out1/1

== system Simple_Model_Packaging_7/信道模型封装/NosieGen/干扰源/If Action Subsystem4 ==
  Input : Inport
  Action Port : ActionPort  ActionPortLabel=case [ 5 ]:
  Out1 : Outport
  wires:
  Input/1 -> Out1/1

== system Simple_Model_Packaging_7/信道模型封装/NosieGen/干扰源/If Action Subsystem5 ==
  In1 : Inport
  Action Port : ActionPort  ActionPortLabel=case [ 0 ]:
  Out1 : Outport
  wires:
  In1/1 -> Out1/1

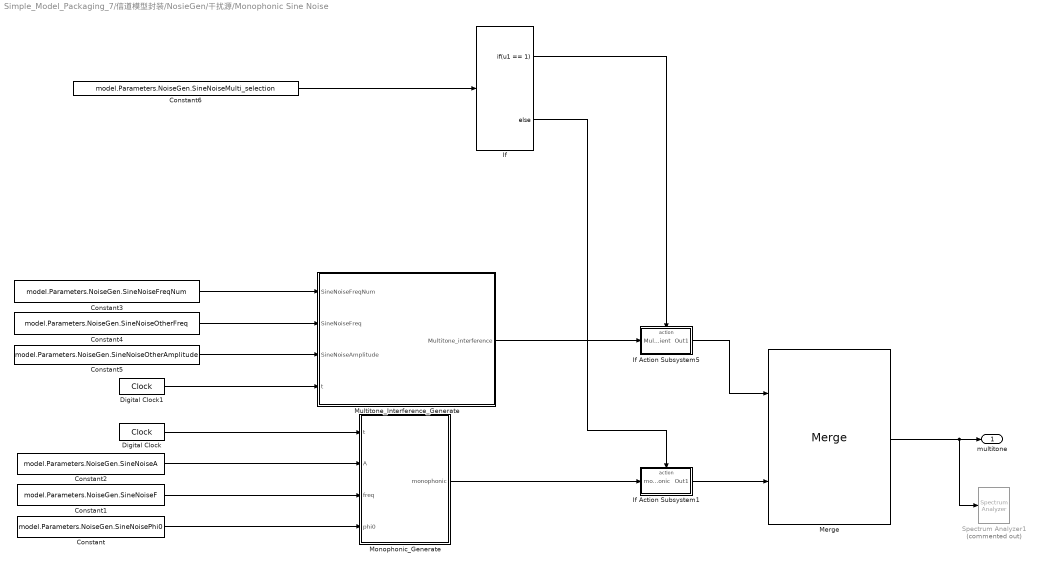
== system Simple_Model_Packaging_7/信道模型封装/NosieGen/干扰源/Monophonic Sine Noise ==
  Constant : Constant  Value=model.Parameters.NoiseGen.SineNoisePhi0
  Constant1 : Constant  Value=model.Parameters.NoiseGen.SineNoiseF
  Constant2 : Constant  Value=model.Parameters.NoiseGen.SineNoiseA
  Constant3 : Constant  Value=model.Parameters.NoiseGen.SineNoiseFreqNum
  Constant4 : Constant  Value=model.Parameters.NoiseGen.SineNoiseOtherFreq
  Constant5 : Constant  Value=model.Parameters.NoiseGen.SineNoiseOtherAmplitude
  Constant6 : Constant  Value=model.Parameters.NoiseGen.SineNoiseMulti_selection
  Digital Clock : DigitalClock  SampleTime=model.Parameters.NoiseGen.NoiseTs
  Digital Clock1 : DigitalClock  SampleTime=model.Parameters.NoiseGen.NoiseTs
  If : If  IfExpression=u1 == 1
  If Action Subsystem1 : Subsystem  TreatAsAtomicUnit=on
  If Action Subsystem5 : Subsystem  TreatAsAtomicUnit=on
  Merge : Merge
  Monophonic_Generate : MATLAB Function  TreatAsAtomicUnit=on
  Multitone_Interference_Generate : MATLAB Function  TreatAsAtomicUnit=on
  Spectrum Analyzer1 : SpectrumAnalyzer  Commented=on  WindowPosition=[-1168 236 916 450]  SampleRate=340000000  AxesScaling=Manual  Span=340000000  StartFrequency=-170000000  StopFrequency=170000000  AveragingMethod=Exponential  YLimits=[-88.119268432802542179,31.5056137623361181]  AllowFFTLengthLessThanSamplesPerUpdate=on
  multitone : Outport
  wires:
  Digital Clock/1 -> Monophonic_Generate/1(t)
  Constant/1 -> Monophonic_Generate/4(phi0)
  Constant2/1 -> Monophonic_Generate/2(A)
  Constant1/1 -> Monophonic_Generate/3(freq)
  Constant3/1 -> Multitone_Interference_Generate/1(SineNoiseFreqNum)
  Constant4/1 -> Multitone_Interference_Generate/2(SineNoiseFreq)
  Constant5/1 -> Multitone_Interference_Generate/3(SineNoiseAmplitude)
  Multitone_Interference_Generate/1(Multitone_interference) -> If Action Subsystem5/1(Multitone_multiplicative_coefficient)
  Merge/1 -> Spectrum Analyzer1/1, multitone/1
  Digital Clock1/1 -> Multitone_Interference_Generate/4(t)
  Constant6/1 -> If/1
  If/1 -> If Action Subsystem5/Action
  If/2 -> If Action Subsystem1/Action
  If Action Subsystem5/1(Out1) -> Merge/1
  Monophonic_Generate/1(monophonic) -> If Action Subsystem1/1(monophonic)
  If Action Subsystem1/1(Out1) -> Merge/2

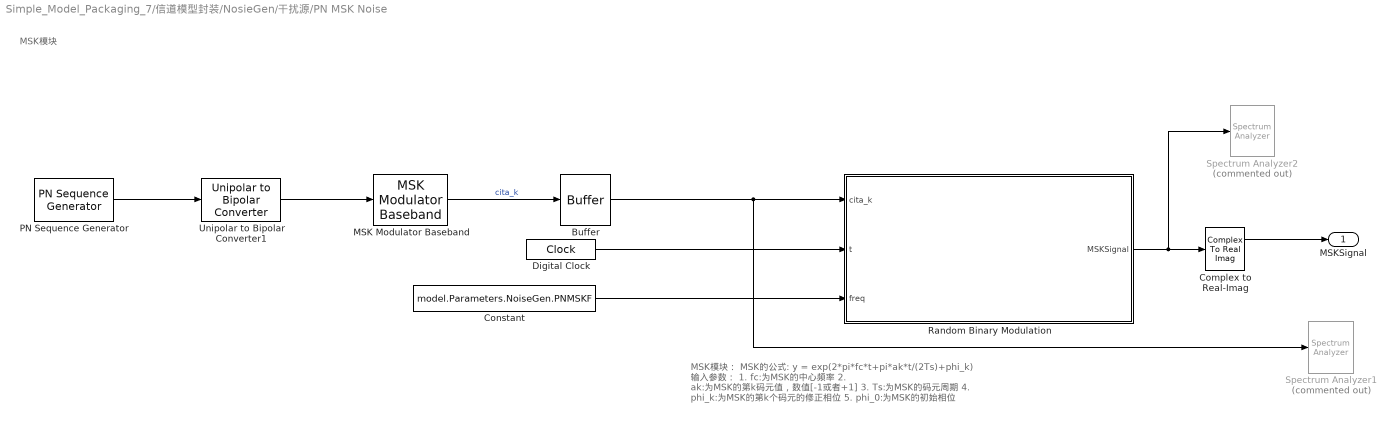
== system Simple_Model_Packaging_7/信道模型封装/NosieGen/干扰源/PN MSK Noise ==
  note: MSK模块
  note: MSK模块：
      | MSK的公式: y = exp(2*pi*fc*t+pi*ak*t/(2Ts)+phi_k)
      | 输入参数：
      | 1. fc:为MSK的中心频率
      | 2. ak:为MSK的第k码元值，数值[-1或者+1]
      | 3. Ts:为MSK的码元周期
      | 4. phi_k:为MSK的第k个码元的修正相位
      | 5. phi_0:为MSK的初始相位
  Buffer : Buffer  N=1  OutputFrames=off
  Complex to Real-Imag : ComplexToRealImag
  Constant : Constant  Value=model.Parameters.NoiseGen.PNMSKF
  Digital Clock : DigitalClock  SampleTime=model.Parameters.NoiseGen.NoiseTs
  MSK Modulator Baseband : commdigbbndcpm2/MSK Modulator Baseband  inputType=Integer  phaseOffset=model.Parameters.NoiseGen.PNMSKPhi0  samplesPerSymbol=model.Parameters.NoiseGen.PNMSKM  RateOptions=Enforce single-rate processing  outDataType=double
  PN Sequence Generator : commseqgen3/PN Sequence Generator  poly=model.Parameters.NoiseGen.PNMSKPolynomial  ini_sta=model.Parameters.NoiseGen.PNMSKInitialstate  outBitMaskSource=Dialog parameter  shift=0  outVarSiz=off  maxOutSizeMode=Dialog parameter  maxOutSize=[10 1]  Ts=model.Parameters.NoiseGen.PNMSKM * model.Parameters.NoiseGen.NoiseTs  sampPerFrame=1  reset=off  bitPackedOutputs=off  outDataType=double  numPackedBits=8  bitPackDataSigned=off  bitPackedOutDType=double
      settings: LibrarySourceBlock=|
      | commhdlsource/PN Sequence
      | Generator
  Random Binary Modulation : MATLAB Function  TreatAsAtomicUnit=on
  Spectrum Analyzer1 : SpectrumAnalyzer  Commented=on  WindowPosition=[-1919 49 1920 954]  SampleRate=340000000  AxesScaling=Manual  Span=340000000  StartFrequency=-170000000  StopFrequency=170000000  AveragingMethod=Exponential  YLimits=[-53.217557687415251166,26.779990315993849492]  AllowFFTLengthLessThanSamplesPerUpdate=on
  Spectrum Analyzer2 : SpectrumAnalyzer  Commented=on  WindowPosition=[-130 -207 1920 954]  SampleRate=340000000  AxesScaling=Manual  Span=340000000  StartFrequency=-170000000  StopFrequency=170000000  AveragingMethod=Exponential  YLimits=[-53.217557687415251166,26.779990315993849492]  AllowFFTLengthLessThanSamplesPerUpdate=on
  Unipolar to Bipolar Converter1 : commutil2/Unipolar to Bipolar Converter  M=2  polarity=Positive  dataType=Inherit via internal rule
  MSKSignal : Outport  OutDataTypeStr=double
  wires:
  Digital Clock/1 -> Random Binary Modulation/2(t)
  Unipolar to Bipolar Converter1/1 -> MSK Modulator Baseband/1
  PN Sequence Generator/1 -> Unipolar to Bipolar Converter1/1
  Constant/1 -> Random Binary Modulation/3(freq)
  MSK Modulator Baseband/1 -> Buffer/1  "cita_k"
  Buffer/1 -> Spectrum Analyzer1/1, Random Binary Modulation/1(cita_k)
  Random Binary Modulation/1(MSKSignal) -> Spectrum Analyzer2/1, Complex to Real-Imag/1
  Complex to Real-Imag/1 -> MSKSignal/1

== system Simple_Model_Packaging_7/信道模型封装/NosieGen/干扰源/Random Binary Noise ==
  note: 此处注意速率转换的整数倍设置
  note: 改模块采用的是概率为贝努利分布的随机二进制数，随机二元码调制噪声的公式如下：
      | Jt = Am*Jn*cos(2*pi*fj*t+phi0)
      | 本质上是数字调相信号，相位翻转180°
  note: 随机二进制调制噪声
  Bernoulli Binary Generator2 : commrandsrc3/Bernoulli Binary Generator  ProbabilityOfZero=model.Parameters.NoiseGen.RandBFZero  SeedSource=Auto  Seed=0  SampleTime=model.Parameters.NoiseGen.PRCodeTs  SamplesPerFrame=1  OutputDataType=double  SimulateUsing=Interpreted execution
  Constant : Constant  Value=model.Parameters.NoiseGen.RandBPFA
  Constant1 : Constant  Value=model.Parameters.NoiseGen.RandBPFF
  Constant2 : Constant  Value=model.Parameters.NoiseGen.RandBPFPhi0
  Digital Clock : DigitalClock  SampleTime=model.Parameters.NoiseGen.NoiseTs
  Random Binary Modulation : MATLAB Function  TreatAsAtomicUnit=on
  Rate Transition : RateTransition  Integrity=off  OutPortSampleTime=model.Parameters.NoiseGen.NoiseTs
  Unipolar to bipolar : MATLAB Function  TreatAsAtomicUnit=on
  Jt : Outport
  wires:
  Random Binary Modulation/1(Jt) -> Jt/1
  Digital Clock/1 -> Random Binary Modulation/2(t)
  Constant/1 -> Random Binary Modulation/3(A)
  Constant1/1 -> Random Binary Modulation/4(freq)
  Constant2/1 -> Random Binary Modulation/5(phi0)
  Rate Transition/1 -> Random Binary Modulation/1(Jn)
  Unipolar to bipolar/1(Jn) -> Rate Transition/1
  Bernoulli Binary Generator2/1 -> Unipolar to bipolar/1(u)

== system Simple_Model_Packaging_7/信道模型封装/NosieGen/干扰源/Subsystem ==
  Band-Limited White Noise : simulink/Sources/Band-Limited White Noise  Cov=model.Parameters.NoiseGen.RFNoisePower  Ts=model.Parameters.NoiseGen.NoiseTs  seed=model.Parameters.NoiseGen.RFNoiseSeed
  Filter : dsparch4/Biquad Filter  Tag=BlockMethodSubSystem  FilterSource=Filter object  CoeffSource=Specify via dialog  FilterObject=model.Parameters.NoiseGen.RFNoiseFilterObj  IIRFiltStruct=Direct form II  BiQuadCoeffs=[1 2 1 1 -1.48178412853867569 0.831585910854089061;1 2 1 1 -1.27721148327892942 0.578720214976092495;1 2 1 1 -1.14298050253990113 0.412801598096188771;1 2 1 1 -1.06189684687510177 0.31257668783031084;1 2 1 1 -1.02371666858405952 0.265383392069520774]  ScaleValues=[0.0874504455788533558;0.0753771829242907976;0.0674552738890718956;0.0626699602388022664;0.0604166808713653344;1]  IC=0  ICnum=0  ICden=0  a0Flag=Warning  optimizeScaleValues=on  ScaleValueMode=Specify via input port (g)  roundingMode=Floor  overflowMode=off  scaleValueFracLength=14  denProdOutputFracLength=30  denAccumFracLength=30  secondMemoryFracLength=15
  Input : Outport
  wires:
  Band-Limited White Noise/1 -> Filter/1
  Filter/1 -> Input/1

== system Simple_Model_Packaging_7/信道模型封装/NosieGen/调制方式/AM ==
  Jammer Source : Inport
  AM_Carrier : MATLAB Function  TreatAsAtomicUnit=on
  Constant : Constant  Value=model.Parameters.NoiseGen.Modulator.AMA
  Constant1 : Constant  Value=model.Parameters.NoiseGen.Modulator.AMF
  Constant2 : Constant  Value=model.Parameters.NoiseGen.Modulator.Ma
  Digital Clock : DigitalClock  SampleTime=model.Parameters.NoiseGen.NoiseTs
  AM_Signal : Outport
  wires:
  Digital Clock/1 -> AM_Carrier/1(t)
  AM_Carrier/1(y) -> AM_Signal/1  "ChirpSignal"
  Constant2/1 -> AM_Carrier/5(Ma)
  Constant1/1 -> AM_Carrier/3(freq)
  Constant/1 -> AM_Carrier/2(A)
  Jammer Source/1 -> AM_Carrier/4(carrier_low_freq)

== system Simple_Model_Packaging_7/信道模型封装/NosieGen/调制方式/FM ==
  InputSignal : Inport
  Constant : Constant  Value=model.Parameters.NoiseGen.Modulator.FMA
  Constant1 : Constant  Value=model.Parameters.NoiseGen.Modulator.FMF
  Constant2 : Constant  Value=model.Parameters.NoiseGen.Modulator.FMPhi0
  Constant3 : Constant  Value=model.Parameters.NoiseGen.Modulator.FMK
  Digital Clock : DigitalClock  SampleTime=model.Parameters.NoiseGen.NoiseTs
  MATLAB Function : MATLAB Function  TreatAsAtomicUnit=on
  FM_Signal : Outport
  wires:
  Digital Clock/1 -> MATLAB Function/1(t)
  MATLAB Function/1(y) -> FM_Signal/1
  InputSignal/1 -> MATLAB Function/2(signal)
  Constant/1 -> MATLAB Function/3(A)
  Constant1/1 -> MATLAB Function/4(freq)
  Constant2/1 -> MATLAB Function/5(phi0)
  Constant3/1 -> MATLAB Function/6(K)

== system Simple_Model_Packaging_7/信道模型封装/NosieGen/调制方式/If Action Subsystem3 ==
  Jammer Source : Inport
  Action Port : ActionPort  ActionPortLabel=default:
  Constant : Constant  Value=0
  Real-Imag to Complex : RealImagToComplex
  Out1 : Outport
  wires:
  Constant/1 -> Real-Imag to Complex/2
  Jammer Source/1 -> Real-Imag to Complex/1
  Real-Imag to Complex/1 -> Out1/1

== system Simple_Model_Packaging_7/信道模型封装/NosieGen/调制方式/If Action Subsystem4 ==
  AM_Signal : Inport
  Action Port : ActionPort  ActionPortLabel=case [ 1 ]:
  Constant : Constant  Value=0
  Real-Imag to Complex : RealImagToComplex
  Out1 : Outport
  wires:
  Constant/1 -> Real-Imag to Complex/2
  AM_Signal/1 -> Real-Imag to Complex/1
  Real-Imag to Complex/1 -> Out1/1

== system Simple_Model_Packaging_7/信道模型封装/NosieGen/调制方式/If Action Subsystem5 ==
  PM_Signal : Inport
  Action Port : ActionPort  ActionPortLabel=case [ 2 ]:
  Constant : Constant  Value=0
  Real-Imag to Complex : RealImagToComplex
  Out1 : Outport
  wires:
  Constant/1 -> Real-Imag to Complex/2
  PM_Signal/1 -> Real-Imag to Complex/1
  Real-Imag to Complex/1 -> Out1/1

== system Simple_Model_Packaging_7/信道模型封装/NosieGen/调制方式/If Action Subsystem6 ==
  FM_Signal : Inport
  Action Port : ActionPort  ActionPortLabel=case [ 3 ]:
  Constant : Constant  Value=0
  Real-Imag to Complex : RealImagToComplex
  Out1 : Outport
  wires:
  Constant/1 -> Real-Imag to Complex/2
  FM_Signal/1 -> Real-Imag to Complex/1
  Real-Imag to Complex/1 -> Out1/1

== system Simple_Model_Packaging_7/信道模型封装/NosieGen/调制方式/PM ==
  InputSignal : Inport
  Constant : Constant  Value=model.Parameters.NoiseGen.Modulator.PMA
  Constant1 : Constant  Value=model.Parameters.NoiseGen.Modulator.PMF
  Constant2 : Constant  Value=model.Parameters.NoiseGen.Modulator.PMPhi0
  Constant3 : Constant  Value=model.Parameters.NoiseGen.Modulator.PMK
  Digital Clock : DigitalClock  SampleTime=model.Parameters.NoiseGen.NoiseTs
  MATLAB Function : MATLAB Function  TreatAsAtomicUnit=on
  PM_Signal : Outport
  wires:
  Digital Clock/1 -> MATLAB Function/1(t)
  InputSignal/1 -> MATLAB Function/2(signal)
  MATLAB Function/1(y) -> PM_Signal/1
  Constant/1 -> MATLAB Function/3(A)
  Constant1/1 -> MATLAB Function/4(freq)
  Constant3/1 -> MATLAB Function/5(K)
  Constant2/1 -> MATLAB Function/6(phi0)

== system Simple_Model_Packaging_7/信道模型封装/NosieGen/干扰方式/ChirpBasebandSignalGenerate/Frequency_Check ==
  ChirpSignal : Inport
  Derivative : Derivative
  Phase Extractor : dspsigops/Phase Extractor  TreatFramesIndependently=off  SimulateUsing=Code generation
  FrequencyConversionLine : Outport
  wires:
  ChirpSignal/1 -> Phase Extractor/1
  Phase Extractor/1 -> Derivative/1
  Derivative/1 -> FrequencyConversionLine/1

== system Simple_Model_Packaging_7/信道模型封装/NosieGen/干扰源/Monophonic Sine Noise/If Action Subsystem1 ==
  monophonic : Inport
  Action Port : ActionPort  ActionPortLabel=else
  Out1 : Outport
  wires:
  monophonic/1 -> Out1/1

== system Simple_Model_Packaging_7/信道模型封装/NosieGen/干扰源/Monophonic Sine Noise/If Action Subsystem5 ==
  Multitone_multiplicative_coefficient : Inport
  Action Port : ActionPort  ActionPortLabel=if(u1 == 1)
  Out1 : Outport
  wires:
  Multitone_multiplicative_coefficient/1 -> Out1/1

== matlab function Simple_Model_Packaging_7/信道模型封装/NosieGen/干扰源/Random Binary Noise/Unipolar to bipolar ==
  data: u input; Jn output
function Jn= fcn(u)
    Jn = 2*u-1;
end

== matlab function Simple_Model_Packaging_7/信道模型封装/NosieGen/调制方式/AM/AM_Carrier ==
  data: y output; t input; A input; freq input; carrier_low_freq input; Ma input
function y = AM_Carrier(t, A, freq, carrier_low_freq, Ma)
    y = A*(1+Ma*carrier_low_freq)*cos(2*pi*freq*t);
end

== matlab function Simple_Model_Packaging_7/信道模型封装/NosieGen/调制方式/FM/MATLAB Function ==
  data: t input; signal input; y output; A input; freq input; phi0 input; K input
function y = FM(t, signal, A, freq, phi0, K)
   y = A*cos(2*pi*(freq+K*signal)*t+phi0) ;
end

== matlab function Simple_Model_Packaging_7/信道模型封装/NosieGen/多频干扰/MultiFreq/MATLAB Function1 ==
  data: y output; t input; f input
% function y = carrierGenerator(t)
%     fc = 5e6;
%     y = exp(1i*2*pi*fc*t);

function y = carrierGenerator(t, f)
    y = exp(1i*2*pi*f*t);
end
